simulink model "modfivecounter"  (R2020a)
settings: Solver=VariableStepAuto  StartTime=0.0  StopTime=10.0  RelTol=1e-3
settings Model: Creator=Admin  LastModifiedBy=Admin

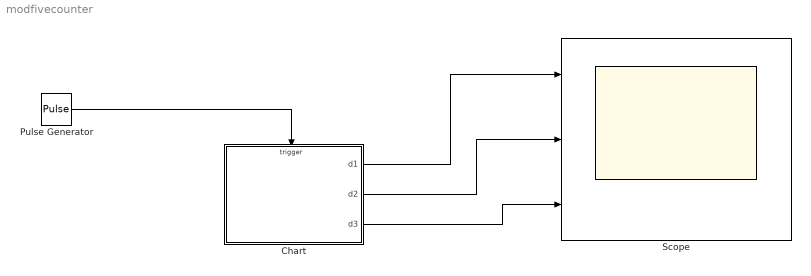
== system modfivecounter ==
  Chart : Stateflow chart  TreatAsAtomicUnit=on
  Pulse Generator : DiscretePulseGenerator  PulseType=Time based  Period=0.1  PulseWidth=5
  Scope : Scope  NumInputPorts=3
  wires:
  Pulse Generator/1 -> Chart/Trigger
  Chart/1(d1) -> Scope/1
  Chart/2(d2) -> Scope/2
  Chart/3(d3) -> Scope/3

== stateflow chart modfivecounter/Chart ==
  state Digit1 [parallel]
    settings: executionOrder=1
    state One
      en:
      d1=1;
    state Two
      en:
      d1=2;
    state Zero
      en:
      d1=0;
    state Three
      en:
      d1=3;
    state Four
      en:
      d1=4;
    Digit1.Two -> Digit1.Three : InputClick
    Digit1.Zero -> Digit1.One : InputClick
    Digit1.One -> Digit1.Two : InputClick
    (default) -> Digit1.Zero
    Digit1.Four -> Digit1.Zero : InputClick/{Click2}
    Digit1.Three -> Digit1.Four : InputClick
  state Digit2 [parallel]
    settings: executionOrder=2
    state One
      en:
      d2=1;
    state Two
      en:
      d2=2;
    state Zero
      en:
      d2=0;
    state Three
      en:
      d2=3;
    state Four
      en:
      d2=4;
    Digit2.Two -> Digit2.Three : Click2
    Digit2.Zero -> Digit2.One : Click2
    Digit2.One -> Digit2.Two : Click2
    (default) -> Digit2.Zero
    Digit2.Four -> Digit2.Zero : Click2/{Click3}
    Digit2.Three -> Digit2.Four : Click2
  state Digit3 [parallel]
    settings: executionOrder=3
    state One
      en:
      d2=1;
    state Two
      en:
      d3=2;
    state Zero
      en:
      d3=0;
    state Three
      en:
      d3=3;
    state Four
      en:
      d3=4;
    Digit3.Two -> Digit3.Three : Click3
    Digit3.Zero -> Digit3.One : Click3
    Digit3.One -> Digit3.Two : Click3
    (default) -> Digit3.Zero
    Digit3.Four -> Digit3.Zero : Click3
    Digit3.Three -> Digit3.Four : Click3
  (default) -> Digit1
  data: d1 output; d2 output; d3 output
  events: InputClick input RISING_EDGE_EVENT; Click2 local FUNCTION_CALL_EVENT; Click3 local FUNCTION_CALL_EVENT
